simulink model "BatteryController_Rev1"  (Simulink 7.7)
settings: Solver=FixedStepDiscrete  StartTime=0.0  StopTime=10.0  RelTol=1e-3
PreLoadFcn:
  | try, eval([bdroot '_setup']); catch, eval('model_setup', ''); end
InitFcn:
  | try, eval([bdroot '_setup']); catch, eval('model_setup', ''); end
undefined symbols (not defined in the file or in its folder): ECU555, motohawk_build_version, motohawk_trunc_name, motohawk_vardec_path
libraries: MotoHawk_lib x213, motohawk_annotations_lib x6, motohawk_control_primitives_lib x2, simulink x1
(part 4 of 4)

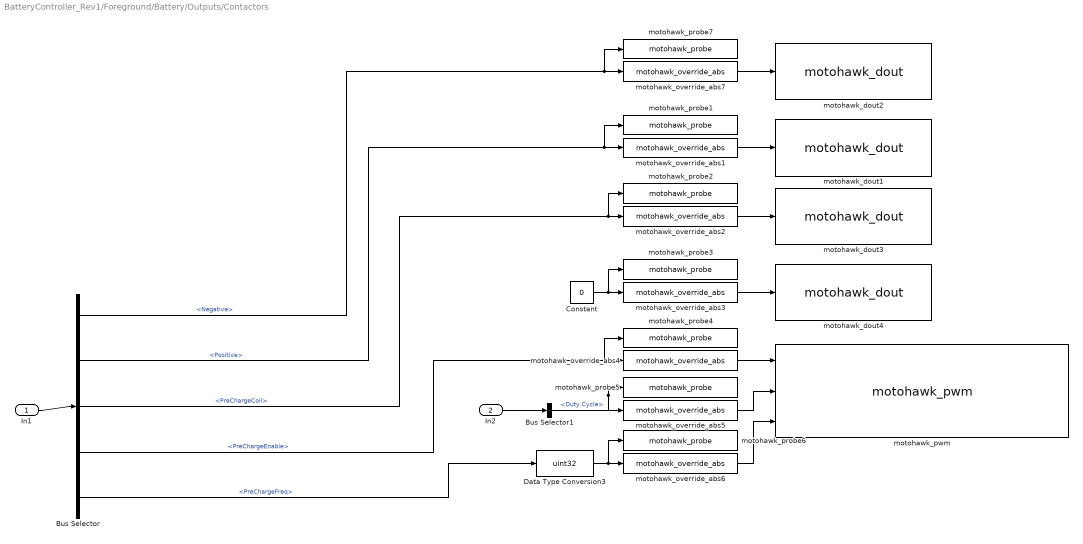
== system BatteryController_Rev1/Foreground/Battery/Outputs/Contactors ==
  In1 : Inport
  In2 : Inport  Port=2
  Bus Selector : BusSelector  OutputSignals=Battery States.Contactors.Negative,Battery States.Contactors.Positive,Battery States.Contactors.PreChargeCoil,Battery States.Contactors.PreChargeEnable,Battery States.Contactors.PreChargeFreq
  Bus Selector1 : BusSelector  OutputSignals=Contactors.Duty Cycle
  Constant : Constant  Value=0  OutDataTypeStr=boolean
  Data Type Conversion3 : DataTypeConversion  OutDataTypeStr=uint32
  motohawk_dout1 : MotoHawk_lib/Digital I//O Blocks/motohawk_dout  resource_name=[]  text_resource=FUEL 2  target=ECU555-48-0707  use_diag=off  use_vardec=off  nam='DOUT'  read_level=1  write_level=1  group='System | I/O Pins | Outputs Config'
  motohawk_dout2 : MotoHawk_lib/Digital I//O Blocks/motohawk_dout  resource_name=[]  text_resource=FUEL 1  target=ECU555-48-0707  use_diag=off  use_vardec=off  nam='DOUT'  read_level=1  write_level=1  group='System | I/O Pins | Outputs Config'
  motohawk_dout3 : MotoHawk_lib/Digital I//O Blocks/motohawk_dout  resource_name=[]  text_resource=FUEL 3  target=ECU555-48-0707  use_diag=off  use_vardec=off  nam='DOUT'  read_level=1  write_level=1  group='System | I/O Pins | Outputs Config'
  motohawk_dout4 : MotoHawk_lib/Digital I//O Blocks/motohawk_dout  resource_name=[]  text_resource=FUEL 4  target=ECU555-48-0707  use_diag=off  use_vardec=off  nam='DOUT'  read_level=1  write_level=1  group='System | I/O Pins | Outputs Config'
  motohawk_override_abs1 : MotoHawk_lib/Calibration & Probing Blocks/motohawk_override_abs  SystemSampleTime=-1  parent_name='Coil1_Pos_Ovr'  parent_val=0  show_more=on  name_source=Use Parameter  parent_read_level=1  parent_override_level=1  view_as=Number  enum_struct={'Disabled', 'Enabled'}  use_help_units=off  parent_help=''  parent_units=''  use_min_max=off  parent_min=-inf  parent_max=inf  use_precision=off  parent_precision=''  parent_gain=1  parent_offset=0  parent_exp=1  use_mototune_group=off  parent_group=motohawk_vardec_path(gcb)
  motohawk_override_abs2 : MotoHawk_lib/Calibration & Probing Blocks/motohawk_override_abs  SystemSampleTime=-1  parent_name='Coil2_Pos_Ovr'  parent_val=0  show_more=on  name_source=Use Parameter  parent_read_level=1  parent_override_level=1  view_as=Number  enum_struct={'Disabled', 'Enabled'}  use_help_units=off  parent_help=''  parent_units=''  use_min_max=off  parent_min=-inf  parent_max=inf  use_precision=off  parent_precision=''  parent_gain=1  parent_offset=0  parent_exp=1  use_mototune_group=off  parent_group=motohawk_vardec_path(gcb)
  motohawk_override_abs3 : MotoHawk_lib/Calibration & Probing Blocks/motohawk_override_abs  SystemSampleTime=-1  parent_name='Coil3_Pos_Ovr'  parent_val=0  show_more=on  name_source=Use Parameter  parent_read_level=1  parent_override_level=1  view_as=Number  enum_struct={'Disabled', 'Enabled'}  use_help_units=off  parent_help=''  parent_units=''  use_min_max=off  parent_min=-inf  parent_max=inf  use_precision=off  parent_precision=''  parent_gain=1  parent_offset=0  parent_exp=1  use_mototune_group=off  parent_group=motohawk_vardec_path(gcb)
  motohawk_override_abs4 : MotoHawk_lib/Calibration & Probing Blocks/motohawk_override_abs  SystemSampleTime=-1  parent_name='PreCharge_Enable_Ovr'  parent_val=0  show_more=on  name_source=Use Parameter  parent_read_level=1  parent_override_level=1  view_as=Number  enum_struct={'Disabled', 'Enabled'}  use_help_units=off  parent_help=''  parent_units=''  use_min_max=off  parent_min=-inf  parent_max=inf  use_precision=off  parent_precision=''  parent_gain=1  parent_offset=0  parent_exp=1  use_mototune_group=off  parent_group=motohawk_vardec_path(gcb)
  motohawk_override_abs5 : MotoHawk_lib/Calibration & Probing Blocks/motohawk_override_abs  SystemSampleTime=-1  parent_name='PreCharge_Duty_Cyle_Ovr'  parent_val=0  show_more=on  name_source=Use Parameter  parent_read_level=1  parent_override_level=1  view_as=Number  enum_struct={'Disabled', 'Enabled'}  use_help_units=off  parent_help=''  parent_units=''  use_min_max=off  parent_min=-inf  parent_max=inf  use_precision=off  parent_precision=''  parent_gain=1  parent_offset=0  parent_exp=1  use_mototune_group=off  parent_group=motohawk_vardec_path(gcb)
  motohawk_override_abs6 : MotoHawk_lib/Calibration & Probing Blocks/motohawk_override_abs  SystemSampleTime=-1  parent_name='PreCharge_Freq_Ovr'  parent_val=0  show_more=on  name_source=Use Parameter  parent_read_level=1  parent_override_level=1  view_as=Number  enum_struct={'Disabled', 'Enabled'}  use_help_units=off  parent_help=''  parent_units=''  use_min_max=off  parent_min=-inf  parent_max=inf  use_precision=off  parent_precision=''  parent_gain=1  parent_offset=0  parent_exp=1  use_mototune_group=off  parent_group=motohawk_vardec_path(gcb)
  motohawk_override_abs7 : MotoHawk_lib/Calibration & Probing Blocks/motohawk_override_abs  SystemSampleTime=-1  parent_name='Coil1_Neg_Ovr'  parent_val=0  show_more=on  name_source=Use Parameter  parent_read_level=1  parent_override_level=1  view_as=Number  enum_struct={'Disabled', 'Enabled'}  use_help_units=off  parent_help=''  parent_units=''  use_min_max=off  parent_min=-inf  parent_max=inf  use_precision=off  parent_precision=''  parent_gain=1  parent_offset=0  parent_exp=1  use_mototune_group=off  parent_group=motohawk_vardec_path(gcb)
  motohawk_probe1 : MotoHawk_lib/Calibration & Probing Blocks/motohawk_probe  nam='Coil1_Pos_Prb'  show_more=on  name_source=Use Parameter  read_level=1  view_as=Number  enum_struct={'Disabled', 'Enabled'}  vector_style=Wide Row  use_help_units=off  help=''  units=''  use_header_enum=off  row_header_enum={}  col_header_enum={}  use_precision=off  precision=''  gain=1  offset=0  exp=1  use_mototune_group=off  mototune_group=motohawk_vardec_path(gcb)
  motohawk_probe2 : MotoHawk_lib/Calibration & Probing Blocks/motohawk_probe  nam='Coil2_Pos_Prb'  show_more=on  name_source=Use Parameter  read_level=1  view_as=Number  enum_struct={'Disabled', 'Enabled'}  vector_style=Wide Row  use_help_units=off  help=''  units=''  use_header_enum=off  row_header_enum={}  col_header_enum={}  use_precision=off  precision=''  gain=1  offset=0  exp=1  use_mototune_group=off  mototune_group=motohawk_vardec_path(gcb)
  motohawk_probe3 : MotoHawk_lib/Calibration & Probing Blocks/motohawk_probe  nam='Coil3_Pos_Prb'  show_more=on  name_source=Use Parameter  read_level=1  view_as=Number  enum_struct={'Disabled', 'Enabled'}  vector_style=Wide Row  use_help_units=off  help=''  units=''  use_header_enum=off  row_header_enum={}  col_header_enum={}  use_precision=off  precision=''  gain=1  offset=0  exp=1  use_mototune_group=off  mototune_group=motohawk_vardec_path(gcb)
  motohawk_probe4 : MotoHawk_lib/Calibration & Probing Blocks/motohawk_probe  nam='PreCharge_Enable_Prb'  show_more=on  name_source=Use Parameter  read_level=1  view_as=Number  enum_struct={'Disabled', 'Enabled'}  vector_style=Wide Row  use_help_units=off  help=''  units=''  use_header_enum=off  row_header_enum={}  col_header_enum={}  use_precision=off  precision=''  gain=1  offset=0  exp=1  use_mototune_group=off  mototune_group=motohawk_vardec_path(gcb)
  motohawk_probe5 : MotoHawk_lib/Calibration & Probing Blocks/motohawk_probe  nam='PreCharge_Duty_Cycle_Prb'  show_more=on  name_source=Use Parameter  read_level=1  view_as=Number  enum_struct={'Disabled', 'Enabled'}  vector_style=Wide Row  use_help_units=off  help=''  units=''  use_header_enum=off  row_header_enum={}  col_header_enum={}  use_precision=off  precision=''  gain=1  offset=0  exp=1  use_mototune_group=off  mototune_group=motohawk_vardec_path(gcb)
  motohawk_probe6 : MotoHawk_lib/Calibration & Probing Blocks/motohawk_probe  nam='PreCharge_Freq_Prb'  show_more=on  name_source=Use Parameter  read_level=1  view_as=Number  enum_struct={'Disabled', 'Enabled'}  vector_style=Wide Row  use_help_units=off  help=''  units=''  use_header_enum=off  row_header_enum={}  col_header_enum={}  use_precision=off  precision=''  gain=1  offset=0  exp=1  use_mototune_group=off  mototune_group=motohawk_vardec_path(gcb)
  motohawk_probe7 : MotoHawk_lib/Calibration & Probing Blocks/motohawk_probe  nam='Coil1_Neg_Prb'  show_more=on  name_source=Use Parameter  read_level=1  view_as=Number  enum_struct={'Disabled', 'Enabled'}  vector_style=Wide Row  use_help_units=off  help=''  units=''  use_header_enum=off  row_header_enum={}  col_header_enum={}  use_precision=off  precision=''  gain=1  offset=0  exp=1  use_mototune_group=off  mototune_group=motohawk_vardec_path(gcb)
  motohawk_pwm : MotoHawk_lib/Analog I//O Blocks/motohawk_pwm  res_name=[]  text_resource=EST 1  code_resource=NONE  val_resource=-1  target=ECU555-48-0707  resource_enum_str=(None)=-1,FUELP=0,LIAC=7,HORN=8,SPARE=9,FUEL 1=12,FUEL 2=13,FUEL 3=14,FUEL 4=15,TACH=24,EST 1=36,EST 2=37  freq_mode=-1  min_freq=2  use_max_freq=off  max_freq=42949672.96  use_enable=on  use_brake=off  output_current=off  output_fault_status=off  use_child=off  use_vardec=off  nam='PWM'  read_level=1  write_level=1  group='System | I/O Pins | Outputs Config'
  wires:
  motohawk_override_abs7/1 -> motohawk_dout2/1
  motohawk_override_abs1/1 -> motohawk_dout1/1
  motohawk_override_abs6/1 -> motohawk_pwm/3
  motohawk_override_abs5/1 -> motohawk_pwm/2
  motohawk_override_abs4/1 -> motohawk_pwm/1
  motohawk_override_abs3/1 -> motohawk_dout4/1
  motohawk_override_abs2/1 -> motohawk_dout3/1
  Data Type Conversion3/1 -> motohawk_override_abs6/1, motohawk_probe6/1
  Constant/1 -> motohawk_override_abs3/1, motohawk_probe3/1
  In1/1 -> Bus Selector/1
  Bus Selector/1 -> motohawk_override_abs7/1, motohawk_probe7/1  "<Negative>"
  Bus Selector/2 -> motohawk_override_abs1/1, motohawk_probe1/1  "<Positive>"
  Bus Selector/3 -> motohawk_override_abs2/1, motohawk_probe2/1  "<PreChargeCoil>"
  Bus Selector/4 -> motohawk_override_abs4/1, motohawk_probe4/1  "<PreChargeEnable>"
  Bus Selector/5 -> Data Type Conversion3/1  "<PreChargeFreq>"
  In2/1 -> Bus Selector1/1
  Bus Selector1/1 -> motohawk_override_abs5/1, motohawk_probe5/1  "<Duty Cycle>"

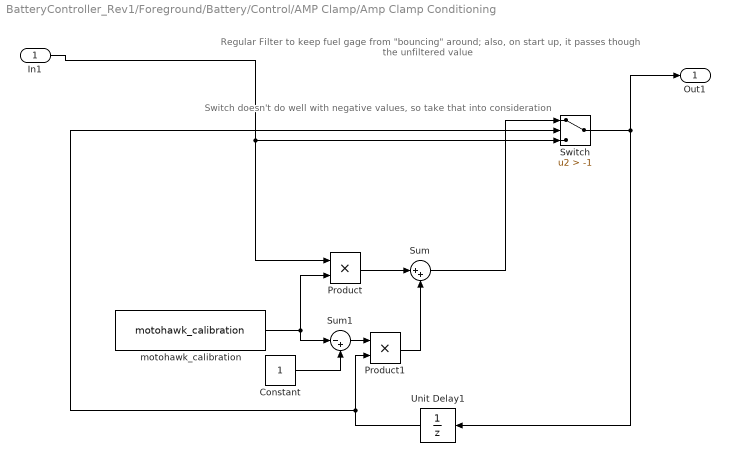
== system BatteryController_Rev1/Foreground/Battery/Control/AMP Clamp/Amp Clamp Conditioning ==
  note: Regular Filter to keep fuel gage from "bouncing" around;
      | also, on start up, it passes though the unfiltered value
  note: Switch doesn't do well with negative values,
      | so take that into consideration
  In1 : Inport
  Constant : Constant
  Product : Product  RndMeth=Zero
  Product1 : Product  RndMeth=Zero
  Sum : Sum  Inputs=|++
  Sum1 : Sum  Inputs=|-+
  Switch : Switch  Criteria=u2 > Threshold  Threshold=-1
  Unit Delay1 : UnitDelay  X0=-1  SampleTime=-1
  motohawk_calibration : MotoHawk_lib/Calibration & Probing Blocks/motohawk_calibration  nam='Amp_Clamp_K'  val=.001  storage=Calibration NV  show_more=on  name_source=Use Parameter  data_type=Inherit from 'Default Value'  read_level=1  write_level=1  ovr_cals=on  view_as=Number  enum_struct={'Disabled', 'Enabled'}  vector_style=Wide Row  use_help_units=off  help=''  units=''  use_header_enum=off  row_header_enum={}  col_header_enum={}  use_min_max=on  min_val=0  max_val=1  use_precision=on  precision='1.4'  gain=1  offset=0  exp=1  use_mototune_group=off  mototune_group=motohawk_vardec_path(gcb)
  Out1 : Outport
  wires:
  motohawk_calibration/1 -> Product/2, Sum1/1
  Product/1 -> Sum/1
  Constant/1 -> Sum1/2
  Sum1/1 -> Product1/1
  Product1/1 -> Sum/2
  Unit Delay1/1 -> Product1/2, Switch/2
  Sum/1 -> Switch/1
  Switch/1 -> Out1/1, Unit Delay1/1
  In1/1 -> Product/1, Switch/3

== system BatteryController_Rev1/Foreground/Battery/Control/Battery States/Delay3 ==
  Enable : EnablePort
  Delay 3 Chart : Stateflow chart  TreatAsAtomicUnit=on
  motohawk_calibration2 : MotoHawk_lib/Calibration & Probing Blocks/motohawk_calibration  nam='Delay_3_Cal'  val=60  storage=Calibration  show_more=on  name_source=Use Parameter  data_type=double  read_level=1  write_level=1  ovr_cals=on  view_as=Number  enum_struct={'Disabled', 'Enabled'}  vector_style=Wide Row  use_help_units=off  help=''  units=''  use_header_enum=off  row_header_enum={}  col_header_enum={}  use_min_max=off  min_val=-inf  max_val=inf  use_precision=on  precision=''  gain=0.05  offset=0  exp=1  use_mototune_group=off  mototune_group=motohawk_vardec_path(gcb)
  Out1 : Outport
  wires:
  motohawk_calibration2/1 -> Delay 3 Chart/1(delay)
  Delay 3 Chart/1(write) -> Out1/1

== system BatteryController_Rev1/Foreground/Battery/Control/Battery States/Delay5 ==
  Enable : EnablePort
  Delay 5 Chart : Stateflow chart  TreatAsAtomicUnit=on
  motohawk_calibration2 : MotoHawk_lib/Calibration & Probing Blocks/motohawk_calibration  nam='Delay_5_Cal'  val=100  storage=Calibration  show_more=on  name_source=Use Parameter  data_type=double  read_level=1  write_level=1  ovr_cals=on  view_as=Number  enum_struct={'Disabled', 'Enabled'}  vector_style=Wide Row  use_help_units=off  help=''  units=''  use_header_enum=off  row_header_enum={}  col_header_enum={}  use_min_max=off  min_val=-inf  max_val=inf  use_precision=on  precision=''  gain=0.05  offset=0  exp=1  use_mototune_group=off  mototune_group=motohawk_vardec_path(gcb)
  Out1 : Outport
  wires:
  motohawk_calibration2/1 -> Delay 5 Chart/1(delay)
  Delay 5 Chart/1(write) -> Out1/1

== system BatteryController_Rev1/Foreground/Battery/Control/Battery States/Delays ==
  In1 : Inport
  Data Type Conversion : DataTypeConversion
  Unit Delay{,1..4} (5 alike) : UnitDelay  SampleTime=-1
  Out1 : Outport
  wires:
  In1/1 -> Data Type Conversion/1
  Unit Delay/1 -> Unit Delay1/1
  Unit Delay1/1 -> Unit Delay2/1
  Unit Delay2/1 -> Unit Delay3/1
  Unit Delay3/1 -> Unit Delay4/1
  Unit Delay4/1 -> Out1/1
  Data Type Conversion/1 -> Unit Delay/1

== system BatteryController_Rev1/Foreground/Battery/Control/SOC/SOC Conditioning ==
  note: Regular Filter to keep fuel gage from "bouncing" around;
      | also, on start up, it passes though the unfiltered value
  note: Switch doesn't do well with negative values,
      | so take that into consideration
  In1 : Inport
  Constant : Constant
  Product : Product  RndMeth=Zero
  Product1 : Product  RndMeth=Zero
  Sum : Sum  Inputs=|++
  Sum1 : Sum  Inputs=|-+
  Switch : Switch  Criteria=u2 > Threshold  Threshold=-1
  Unit Delay1 : UnitDelay  X0=-1  SampleTime=-1
  motohawk_calibration : MotoHawk_lib/Calibration & Probing Blocks/motohawk_calibration  nam='SOC_K'  val=.001  storage=Calibration NV  show_more=on  name_source=Use Parameter  data_type=Inherit from 'Default Value'  read_level=1  write_level=1  ovr_cals=on  view_as=Number  enum_struct={'Disabled', 'Enabled'}  vector_style=Wide Row  use_help_units=off  help=''  units=''  use_header_enum=off  row_header_enum={}  col_header_enum={}  use_min_max=on  min_val=0  max_val=1  use_precision=on  precision='1.4'  gain=1  offset=0  exp=1  use_mototune_group=off  mototune_group=motohawk_vardec_path(gcb)
  Out1 : Outport
  wires:
  motohawk_calibration/1 -> Product/2, Sum1/1
  Product/1 -> Sum/1
  Constant/1 -> Sum1/2
  Sum1/1 -> Product1/1
  Product1/1 -> Sum/2
  Unit Delay1/1 -> Product1/2, Switch/2
  Sum/1 -> Switch/1
  Switch/1 -> Out1/1, Unit Delay1/1
  In1/1 -> Product/1, Switch/3

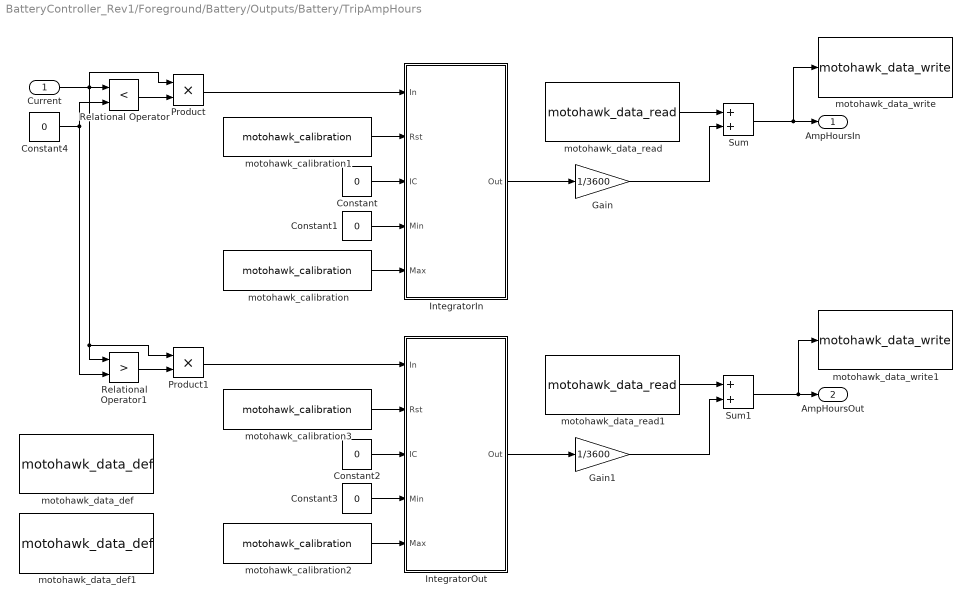
== system BatteryController_Rev1/Foreground/Battery/Outputs/Battery/TripAmpHours ==
  Current : Inport
  Constant{,1..4} (5 alike) : Constant  Value=0
  Gain : Gain  Gain=1/3600
  Gain1 : Gain  Gain=1/3600
  IntegratorIn : Subsystem  AncestorBlock=motohawk_control_primitives_lib/Integrator  mask(Discrete Integrator){samp_time=-1}
      mask prompts: samp_time "Sample Time"
      mask help:
      | Resetable integrator with upper and lower windup limits.
      |
      | If 'Sample Time' is -1, then extra code and RAM will be generated to dynamically calculate dt.
      mask Display:
      | patch([0 0 1 1], 0.75*[0 0.075 0.075 0], [230/255 0/255 0/255])
      | patch([0 0 1 1], 0.75*[0.025 0.05 0.05 0.025], [150/255 0/255 0/255])
      | patch([0 0 1 1], 0.75*[0 0.025 0.025 0], [0/255 0/255 0/255])
      | 
      | disp('\fontsize{16}\bf\it\int dt', 'texmode', 'on')
  IntegratorOut : Subsystem  AncestorBlock=motohawk_control_primitives_lib/Integrator  mask(Discrete Integrator){samp_time=-1}
      mask prompts: samp_time "Sample Time"
      mask help:
      | Resetable integrator with upper and lower windup limits.
      |
      | If 'Sample Time' is -1, then extra code and RAM will be generated to dynamically calculate dt.
      mask Display:
      | patch([0 0 1 1], 0.75*[0 0.075 0.075 0], [230/255 0/255 0/255])
      | patch([0 0 1 1], 0.75*[0.025 0.05 0.05 0.025], [150/255 0/255 0/255])
      | patch([0 0 1 1], 0.75*[0 0.025 0.025 0], [0/255 0/255 0/255])
      | 
      | disp('\fontsize{16}\bf\it\int dt', 'texmode', 'on')
  Product : Product  RndMeth=Zero
  Product1 : Product  RndMeth=Zero
  Relational Operator : RelationalOperator  Operator=<  OutDataTypeStr=boolean
  Relational Operator1 : RelationalOperator  Operator=>  OutDataTypeStr=boolean
  Sum : Sum
  Sum1 : Sum
  motohawk_calibration : MotoHawk_lib/Calibration & Probing Blocks/motohawk_calibration  nam='Max_AmphoursIn'  val=100000  storage=Calibration NV  show_more=off  name_source=Use Parameter  data_type=Inherit from 'Default Value'  read_level=1  write_level=1  ovr_cals=on  view_as=Number  enum_struct={'Disabled', 'Enabled'}  vector_style=Wide Row  use_help_units=off  help=''  units=''  use_header_enum=off  row_header_enum={}  col_header_enum={}  use_min_max=off  min_val=-inf  max_val=inf  use_precision=off  precision=''  gain=1  offset=0  exp=1  use_mototune_group=off  mototune_group=motohawk_vardec_path(gcb)
  motohawk_calibration1 : MotoHawk_lib/Calibration & Probing Blocks/motohawk_calibration  nam='Reset_AmpHoursIn'  val=0  storage=Display NV  show_more=off  name_source=Use Parameter  data_type=Inherit from 'Default Value'  read_level=1  write_level=1  ovr_cals=on  view_as=Number  enum_struct={'Disabled', 'Enabled'}  vector_style=Wide Row  use_help_units=off  help=''  units=''  use_header_enum=off  row_header_enum={}  col_header_enum={}  use_min_max=off  min_val=-inf  max_val=inf  use_precision=off  precision=''  gain=1  offset=0  exp=1  use_mototune_group=off  mototune_group=motohawk_vardec_path(gcb)
  motohawk_calibration2 : MotoHawk_lib/Calibration & Probing Blocks/motohawk_calibration  nam='Max_AmphoursOut'  val=100000  storage=Calibration NV  show_more=off  name_source=Use Parameter  data_type=Inherit from 'Default Value'  read_level=1  write_level=1  ovr_cals=on  view_as=Number  enum_struct={'Disabled', 'Enabled'}  vector_style=Wide Row  use_help_units=off  help=''  units=''  use_header_enum=off  row_header_enum={}  col_header_enum={}  use_min_max=off  min_val=-inf  max_val=inf  use_precision=off  precision=''  gain=1  offset=0  exp=1  use_mototune_group=off  mototune_group=motohawk_vardec_path(gcb)
  motohawk_calibration3 : MotoHawk_lib/Calibration & Probing Blocks/motohawk_calibration  nam='Reset_AmpHoursOut'  val=0  storage=Display NV  show_more=off  name_source=Use Parameter  data_type=Inherit from 'Default Value'  read_level=1  write_level=1  ovr_cals=on  view_as=Number  enum_struct={'Disabled', 'Enabled'}  vector_style=Wide Row  use_help_units=off  help=''  units=''  use_header_enum=off  row_header_enum={}  col_header_enum={}  use_min_max=off  min_val=-inf  max_val=inf  use_precision=off  precision=''  gain=1  offset=0  exp=1  use_mototune_group=off  mototune_group=motohawk_vardec_path(gcb)
  motohawk_data_def : MotoHawk_lib/Data Storage Blocks/motohawk_data_def  nam='AmpIn'  container_nam=''  data=0  typ=double  struct_nam='MyStruct'  storage=NonVolatile  outputRef=off  use_vardec=on  window=Calibration  read_level=1  write_level=1  ovr_cals=on  view_as=Number  enum_struct={'Disabled', 'Enabled'}  vector_style=Wide Row  use_help_units=off  help=''  units=''  use_header_enum=off  row_header_enum=''  col_header_enum=''  use_min_max=off  min_val=-inf  max_val=inf  use_precision=off  precision=''  gain=1  offset=0  exp=1  use_mototune_group=off  mototune_group=motohawk_vardec_path(gcb)  eval_name=MyData  data_stores=motohawk_sfun_data_def_data_stores  struct_instances=motohawk_sfun_data_def_struct_instances  vardecs=motohawk_sfun_data_def_vardecs
  motohawk_data_def1 : MotoHawk_lib/Data Storage Blocks/motohawk_data_def  nam='AmpOut'  container_nam=''  data=0  typ=double  struct_nam='MyStruct'  storage=NonVolatile  outputRef=off  use_vardec=on  window=Calibration  read_level=1  write_level=1  ovr_cals=on  view_as=Number  enum_struct={'Disabled', 'Enabled'}  vector_style=Wide Row  use_help_units=off  help=''  units=''  use_header_enum=off  row_header_enum=''  col_header_enum=''  use_min_max=off  min_val=-inf  max_val=inf  use_precision=off  precision=''  gain=1  offset=0  exp=1  use_mototune_group=off  mototune_group=motohawk_vardec_path(gcb)  eval_name=MyData  data_stores=motohawk_sfun_data_def_data_stores  struct_instances=motohawk_sfun_data_def_struct_instances  vardecs=motohawk_sfun_data_def_vardecs
  motohawk_data_read : MotoHawk_lib/Data Storage Blocks/motohawk_data_read  source=Lookup By Name  structure=Scalar  operation=Read scalar from location by index  sz_vec=4  sz_row=2  sz_col=3  typ=double  nam='AmpIn'  checkNull=on  struct_inst_name='MyData'  struct_nam='MyStruct'
  motohawk_data_read1 : MotoHawk_lib/Data Storage Blocks/motohawk_data_read  source=Lookup By Name  structure=Scalar  operation=Read scalar from location by index  sz_vec=4  sz_row=2  sz_col=3  typ=double  nam='AmpOut'  checkNull=on  struct_inst_name='MyData'  struct_nam='MyStruct'
  motohawk_data_write : MotoHawk_lib/Data Storage Blocks/motohawk_data_write  source=Lookup By Name  structure=Scalar  operation=Write entire data structure at once  sz_vec=9  sz_row=2  sz_col=9  typ=double  nam='AmpIn'  checkNull=on  write_read_only=off  struct_inst_name=''  struct_name='MyStruct'
  motohawk_data_write1 : MotoHawk_lib/Data Storage Blocks/motohawk_data_write  source=Lookup By Name  structure=Scalar  operation=Write entire data structure at once  sz_vec=9  sz_row=2  sz_col=9  typ=double  nam='AmpOut'  checkNull=on  write_read_only=off  struct_inst_name=''  struct_name='MyStruct'
  AmpHoursIn : Outport
  AmpHoursOut : Outport  Port=2
  wires:
  Constant/1 -> IntegratorIn/3(IC)
  Constant1/1 -> IntegratorIn/4(Min)
  motohawk_calibration/1 -> IntegratorIn/5(Max)
  motohawk_calibration1/1 -> IntegratorIn/2(Rst)
  Constant2/1 -> IntegratorOut/3(IC)
  Constant3/1 -> IntegratorOut/4(Min)
  motohawk_calibration2/1 -> IntegratorOut/5(Max)
  motohawk_calibration3/1 -> IntegratorOut/2(Rst)
  Current/1 -> Relational Operator/1, Product/1, Relational Operator1/1, Product1/1
  Constant4/1 -> Relational Operator/2, Relational Operator1/2
  Relational Operator/1 -> Product/2
  Relational Operator1/1 -> Product1/2
  Product/1 -> IntegratorIn/1(In)
  Product1/1 -> IntegratorOut/1(In)
  motohawk_data_read/1 -> Sum/1
  Sum/1 -> AmpHoursIn/1, motohawk_data_write/1
  IntegratorIn/1(Out) -> Gain/1
  motohawk_data_read1/1 -> Sum1/1
  IntegratorOut/1(Out) -> Gain1/1
  Sum1/1 -> AmpHoursOut/1, motohawk_data_write1/1
  Gain/1 -> Sum/2
  Gain1/1 -> Sum1/2

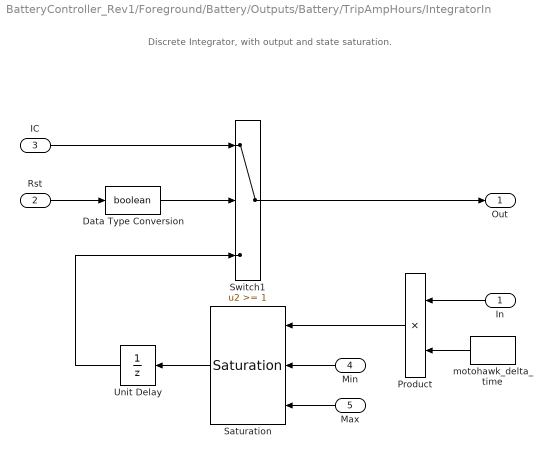
== system BatteryController_Rev1/Foreground/Battery/Outputs/Battery/TripAmpHours/IntegratorIn ==
  note: Discrete Integrator,
      | with output and state saturation.
  In : Inport
  Rst : Inport  Port=2
  IC : Inport  Port=3
  Min : Inport  Port=4
  Max : Inport  Port=5
  Data Type Conversion : DataTypeConversion  OutDataTypeStr=boolean  RndMeth=Zero
  Product : Product  SaturateOnIntegerOverflow=on  InputSameDT=on  OutDataTypeStr=Inherit: Same as first input
  Saturation : motohawk_control_primitives_lib/Saturation  SystemSampleTime=-1
  Switch1 : Switch  Threshold=1  ZeroCross=off  SaturateOnIntegerOverflow=on  InputSameDT=on
  Unit Delay : UnitDelay  SampleTime=-1
  motohawk_delta_time : MotoHawk_lib/Extra Development Blocks/motohawk_delta_time  samp_time=-1  init_val=0  mode=Seconds (double)
  Out : Outport
  wires:
  Switch1/1 -> Out/1
  motohawk_delta_time/1 -> Product/2
  In/1 -> Product/1
  Product/1 -> Saturation/1
  Unit Delay/1 -> Switch1/3
  Rst/1 -> Data Type Conversion/1
  Data Type Conversion/1 -> Switch1/2
  IC/1 -> Switch1/1
  Saturation/1 -> Unit Delay/1
  Min/1 -> Saturation/2
  Max/1 -> Saturation/3

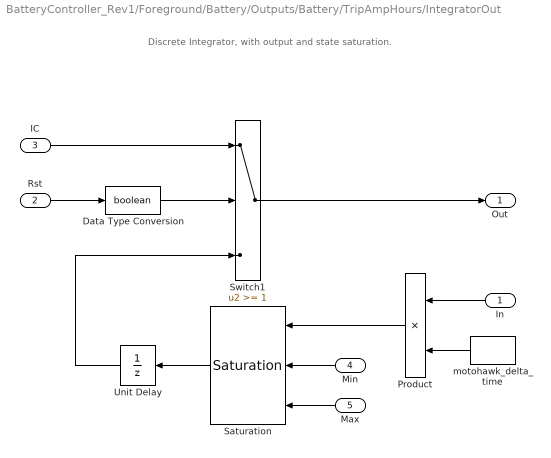
== system BatteryController_Rev1/Foreground/Battery/Outputs/Battery/TripAmpHours/IntegratorOut ==
  note: Discrete Integrator,
      | with output and state saturation.
  In : Inport
  Rst : Inport  Port=2
  IC : Inport  Port=3
  Min : Inport  Port=4
  Max : Inport  Port=5
  Data Type Conversion : DataTypeConversion  OutDataTypeStr=boolean  RndMeth=Zero
  Product : Product  SaturateOnIntegerOverflow=on  InputSameDT=on  OutDataTypeStr=Inherit: Same as first input
  Saturation : motohawk_control_primitives_lib/Saturation  SystemSampleTime=-1
  Switch1 : Switch  Threshold=1  ZeroCross=off  SaturateOnIntegerOverflow=on  InputSameDT=on
  Unit Delay : UnitDelay  SampleTime=-1
  motohawk_delta_time : MotoHawk_lib/Extra Development Blocks/motohawk_delta_time  samp_time=-1  init_val=0  mode=Seconds (double)
  Out : Outport
  wires:
  Switch1/1 -> Out/1
  motohawk_delta_time/1 -> Product/2
  In/1 -> Product/1
  Product/1 -> Saturation/1
  Unit Delay/1 -> Switch1/3
  Rst/1 -> Data Type Conversion/1
  Data Type Conversion/1 -> Switch1/2
  IC/1 -> Switch1/1
  Saturation/1 -> Unit Delay/1
  Min/1 -> Saturation/2
  Max/1 -> Saturation/3

== stateflow chart Foreground/Battery/Control/Battery States/Coil2State ==
  state BatteryDisabled
    during:
    Negative=0;
    Positive=0;
    PreChargeCoil=0;
    PreChargeEnable=0;
    PreChargeFreq=0;
    Freq=0;
  state PreChargeEntry
    entry:
    Freq=FreqStart;
    during:
    Negative=1;
    PreChargeCoil=1;
    PreChargeEnable=1;
    PreChargeFreq=Freq;
    Freq--;
  state BatteryOn
    during:
    Positive=1;
    PreChargeEnable=0;
    PreChargeFreq=0;
    BatteryOn=1;
  state PreChargeNeg
    entry:
    Freq=FreqStart;
    during:
    PreChargeFreq=Freq;
    Freq=Freq-1;
  state PreChargePos
    entry:
    Freq=FreqStart;
    during:
    PreChargeFreq=Freq;
    Freq=Freq+1;
  (default) -> BatteryDisabled
  BatteryDisabled -> PreChargeEntry : [BatteryEnable==1]
  PreChargeEntry -> PreChargePos [order 2] : [FreqStart<=FreqEnd]
  BatteryOn -> BatteryDisabled : [BatteryEnable==0]
  PreChargeEntry -> PreChargeNeg [order 1] : [FreqStart>FreqEnd]
  PreChargeNeg -> BatteryOn : [Freq<=FreqEnd]
  PreChargePos -> BatteryOn : [Freq>=FreqEnd]
  data: Negative output boolean; BatteryEnable input boolean; FreqStart input double; FreqEnd input double; Positive output boolean; PreChargeCoil output boolean; PreChargeEnable output boolean; PreChargeFreq output boolean; Freq local double; BatteryOn output boolean

== stateflow chart Foreground/Battery/Control/AMP Clamp/Amp Clamp Offsets ==
  state default_off
    during: Offset_Out = Offset_In;
  state Offsets
    entry: Offset_Out = Amperage_In;
  state default_on
    during: Offset_Out = Offset_In;
  (default) -> default_off
  default_off -> Offsets : [Connect_Command == 1]
  Offsets -> default_on : [Offset_In == Amperage_In]
  default_on -> default_off : [Connect_Command == 0]
  data: Offset_In input double; Connect_Command input double; Amperage_In input double; Offset_Out output double

== stateflow chart Foreground/Battery/Control/Battery States/Delay5/Delay 5 Chart ==
  state Init
    during: write=0;
  state Counting
    during: count++;
  state Write
    during: write=1;
  state Clear
    during: write=0;
    during: count=0;
  (default) -> Init
  Init -> Counting : [write==0]
  Counting -> Write : [count>=delay]
  Write -> Clear : [write==1]
  Clear -> Init : [write==0]
  data: write output boolean; count local double; delay input double

== stateflow chart Foreground/Battery/Control/SOC/SOC States ==
  state LowAmperage
    during: voltageOut = voltageIn;
    during: currState = 0;
  state HighAmpearge
    during: voltageOut = voltageIn + (amperage * IR);
    during: currState = 1;
  state Counting
    en: tick = 0;
    during: tick++;
    during: voltageOut = voltageIn + (amperage * IR);
    during: currState = 1;
  (default) -> LowAmperage
  LowAmperage -> HighAmpearge : [abs(amperage) >= highAmperage]
  HighAmpearge -> Counting : [abs(amperage) <= lowAmperage]
  Counting -> HighAmpearge [order 2] : [abs(amperage) >= highAmperage]
  Counting -> LowAmperage [order 1] : [tick >= waitTime]
  data: voltageIn input double; voltageOut output double; amperage input double; highAmperage input double; lowAmperage input double; waitTime input int32; currState output double; IR input double; tick local double

== matlab function Foreground/Battery/Control/Battery States/Pack State ==
  data: precharge input double; PackState output double; positive input double
function PackState = fcn(precharge,positive)

if (precharge==0 && positive==0)
    PackState=2; %Disconnected
elseif (precharge==1 && positive==0)
    PackState=3; %Precharging
elseif (precharge==0 && positive==1)
    PackState=4; %Connected-Driving
else
    PackState=1; %Idle (Should never enter state)
end

== stateflow chart Foreground/Battery/Control/Battery States/Precharge State ==
  state Init
    during: state=0;
  state Precharging
    during: state=2;
  state Successful
    during: state=3;
  state Failed
    during: state=4;
  state Wait1
    during: state=2
  state Wait2
    during: state=4;
  state Wait3
    during: state=3;
  state Delay3
    during: delay3Out=1;
  state Delay52
    during: delay5Out=1;
  state Delay51
    during: delay5Out=1;
  Init -> Precharging : [precharge==1]
  Precharging -> Delay3 : [state==2]
  Wait1 -> Failed [order 1] : [current<cal]
  Wait1 -> Successful [order 2] : [current>=cal]
  Delay52 -> Wait3 : [delay5In==1]
  Delay3 -> Wait1 : [delay3In==1]
  Wait2 -> Init : [positive==1]
  Wait3 -> Init : [positive==1]
  (default) -> Init
  Successful -> Delay52 : [state==3]
  Failed -> Delay51 : [state==4]
  Delay51 -> Wait2 : [delay5In==1]
  data: precharge input double; positive input double; current input double; cal input double; state output double; delay3In input boolean; delay3Out output double; delay5In input boolean; delay5Out output double

== matlab function Foreground/Battery/Control/AMP Clamp/Curret Calculation Instantaneos ==
  data: offset input double; curr input double; amps output double; ref input double; sens input double
function amps = fcn(offset,curr,ref,sens)

amps = ((5/ref)*(curr-offset))*(1/sens);

== stateflow chart Foreground/Battery/Control/Battery States/Delay3/Delay 3 Chart ==
  state Init
    during: write=0;
  state Counting
    during: count++;
  state Write
    during: write=1;
  state Clear
    during: write=0;
    during: count=0;
  (default) -> Init
  Init -> Counting : [write==0]
  Counting -> Write : [count>=delay]
  Write -> Clear : [write==1]
  Clear -> Init : [write==0]
  data: write output boolean; count local double; delay input double
